simulink model "windspd"  (R2019b)
settings: Solver=VariableStepAuto  StartTime=0.0  StopTime=10.0  RelTol=1e-3
settings Model: Creator=Chitra Manis Raja  LastModifiedBy=Chitra Manis Raja

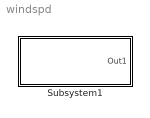
== system windspd ==
  Subsystem1 : Subsystem

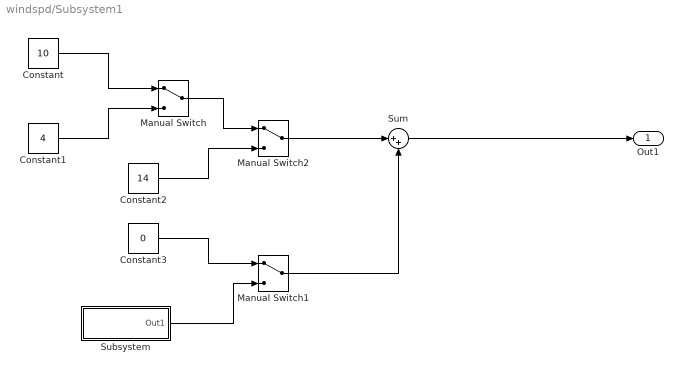
== system windspd/Subsystem1 ==
  Constant : Constant  Value=10
  Constant1 : Constant  Value=4
  Constant2 : Constant  Value=14
  Constant3 : Constant  Value=0
  Manual Switch : ManualSwitch
  Manual Switch1 : ManualSwitch
  Manual Switch2 : ManualSwitch
  Subsystem : Subsystem
  Sum : Sum  Inputs=|++
  Out1 : Outport
  wires:
  Sum/1 -> Out1/1
  Constant3/1 -> Manual Switch1/1
  Constant2/1 -> Manual Switch2/2
  Subsystem/1(Out1) -> Manual Switch1/2
  Manual Switch/1 -> Manual Switch2/1
  Manual Switch1/1 -> Sum/2
  Manual Switch2/1 -> Sum/1
  Constant/1 -> Manual Switch/1
  Constant1/1 -> Manual Switch/2

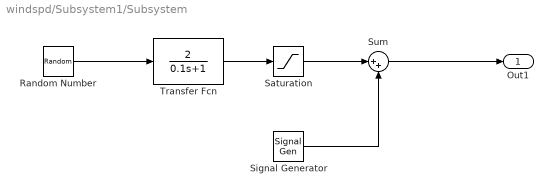
== system windspd/Subsystem1/Subsystem ==
  Random Number : RandomNumber  SampleTime=0.1
  Saturation : Saturate  UpperLimit=3  LowerLimit=-2
  Signal Generator : SignalGenerator  Frequency=0.05  Units=rad/sec
  Sum : Sum  Inputs=|++
  Transfer Fcn : TransferFcn  Numerator=[2]  Denominator=[0.1 1]
  Out1 : Outport
  wires:
  Signal Generator/1 -> Sum/2
  Transfer Fcn/1 -> Saturation/1
  Sum/1 -> Out1/1
  Saturation/1 -> Sum/1
  Random Number/1 -> Transfer Fcn/1
